simulink model "EHB_speedgoat_R2020a_V1"  (R2020a)
settings: Solver=FixedStepDiscrete  StartTime=0.0  StopTime=inf  FixedStep=0.001  RelTol=1e-3  EnableMultiTasking=on
model workspace (MAT data in the model file):
  A : Simulink.Signal (value not decoded)
  B : Simulink.Signal (value not decoded)
  C : Simulink.Signal (value not decoded)
  D : Simulink.Signal (value not decoded)
  E : Simulink.Signal (value not decoded)
  calin = [-9.96 -7.98 -5.98 -3.99 -1.994 0 1.995 3.992 5.99 7.98 9.97]
  calout = [-10 -8 -6 -4 -2 0 2 4 6 8 10]
symbols that are objects in the model workspace (value not decoded): C, D
undefined symbols (not defined in the file): Com1, none, ts_IO612
libraries: simulink x1436, xpcethercatlib x1223, yisutbxlib_utilities x256, xpcutilitieslib x156, hdlsllib x145, canmsglib x46, speedgoatlib_IO602_4 x11, speedgoatlib_IO611 x7, slrttcplib x4, CanManageLib x3, slrtlib x3, xpcseriallib x2
(part 23 of 30)

== system EHB_speedgoat_R2020a_V1/保留/TIF_06/YS4020_M_1/YS4020_M/FIU_CH1 ==
  FIU_SetCH1 : Inport
  "Bit Unpacking " : xpcutilitieslib/Bit Unpacking   SignExtend=on  MaskBitPatterns={[0],[1],[2],[3]}  MaskPackDataType=uint8  MaskPackDataSize=[1]  MaskUnpackDataTypes={'boolean','boolean','boolean','boolean'}  MaskUnpackDataSizes={[1],[1],[1],[1]}
      settings: SourceProductBaseCode=XP
  Bus Creator : BusCreator  Inputs=4
  Protect : Subsystem
  CH1_Out : Outport
  wires:
  FIU_SetCH1/1 -> "Bit Unpacking "/1
  Protect/3(COM_Out) -> Bus Creator/3  "COM_Out"
  Protect/2(KL31_Out) -> Bus Creator/2  "KL31_Out"
  Protect/1(KL30_Out) -> Bus Creator/1  "KL30_Out"
  Protect/4(Open_Out) -> Bus Creator/4  "Open_Out"
  "Bit Unpacking "/1 -> Protect/1(KL30_In)
  "Bit Unpacking "/2 -> Protect/2(KL31_In)
  "Bit Unpacking "/3 -> Protect/3(COM_In)
  "Bit Unpacking "/4 -> Protect/4(Open_In)
  Bus Creator/1 -> CH1_Out/1

== system EHB_speedgoat_R2020a_V1/保留/TIF_06/YS4020_M_1/YS4020_M/FIU_CH10 ==
  FIU_SetCH10 : Inport
  "Bit Unpacking " : xpcutilitieslib/Bit Unpacking   SignExtend=on  MaskBitPatterns={[0],[1],[2],[3]}  MaskPackDataType=uint8  MaskPackDataSize=[1]  MaskUnpackDataTypes={'boolean','boolean','boolean','boolean'}  MaskUnpackDataSizes={[1],[1],[1],[1]}
      settings: SourceProductBaseCode=XP
  Bus Creator : BusCreator  Inputs=4
  Protect : Subsystem
  CH10_Out : Outport
  wires:
  Bus Creator/1 -> CH10_Out/1
  "Bit Unpacking "/4 -> Protect/4(Open_In)
  "Bit Unpacking "/3 -> Protect/3(COM_In)
  "Bit Unpacking "/2 -> Protect/2(KL31_In)
  "Bit Unpacking "/1 -> Protect/1(KL30_In)
  Protect/4(Open_Out) -> Bus Creator/4  "Open_Out"
  Protect/1(KL30_Out) -> Bus Creator/1  "KL30_Out"
  Protect/2(KL31_Out) -> Bus Creator/2  "KL31_Out"
  Protect/3(COM_Out) -> Bus Creator/3  "COM_Out"
  FIU_SetCH10/1 -> "Bit Unpacking "/1

== system EHB_speedgoat_R2020a_V1/保留/TIF_06/YS4020_M_1/YS4020_M/FIU_CH11 ==
  FIU_SetCH1 : Inport
  "Bit Unpacking " : xpcutilitieslib/Bit Unpacking   SignExtend=on  MaskBitPatterns={[0],[1],[2],[3]}  MaskPackDataType=uint8  MaskPackDataSize=[1]  MaskUnpackDataTypes={'boolean','boolean','boolean','boolean'}  MaskUnpackDataSizes={[1],[1],[1],[1]}
      settings: SourceProductBaseCode=XP
  Bus Creator : BusCreator  Inputs=4
  Protect : Subsystem
  CH1_Out : Outport
  wires:
  Bus Creator/1 -> CH1_Out/1
  "Bit Unpacking "/4 -> Protect/4(Open_In)
  "Bit Unpacking "/3 -> Protect/3(COM_In)
  "Bit Unpacking "/2 -> Protect/2(KL31_In)
  "Bit Unpacking "/1 -> Protect/1(KL30_In)
  Protect/4(Open_Out) -> Bus Creator/4  "Open_Out"
  Protect/1(KL30_Out) -> Bus Creator/1  "KL30_Out"
  Protect/2(KL31_Out) -> Bus Creator/2  "KL31_Out"
  Protect/3(COM_Out) -> Bus Creator/3  "COM_Out"
  FIU_SetCH1/1 -> "Bit Unpacking "/1

== system EHB_speedgoat_R2020a_V1/保留/TIF_06/YS4020_M_1/YS4020_M/FIU_CH12 ==
  FIU_SetCH10 : Inport
  "Bit Unpacking " : xpcutilitieslib/Bit Unpacking   SignExtend=on  MaskBitPatterns={[0],[1],[2],[3]}  MaskPackDataType=uint8  MaskPackDataSize=[1]  MaskUnpackDataTypes={'boolean','boolean','boolean','boolean'}  MaskUnpackDataSizes={[1],[1],[1],[1]}
      settings: SourceProductBaseCode=XP
  Bus Creator : BusCreator  Inputs=4
  Protect : Subsystem
  CH10_Out : Outport
  wires:
  FIU_SetCH10/1 -> "Bit Unpacking "/1
  Protect/3(COM_Out) -> Bus Creator/3  "COM_Out"
  Protect/2(KL31_Out) -> Bus Creator/2  "KL31_Out"
  Protect/1(KL30_Out) -> Bus Creator/1  "KL30_Out"
  Protect/4(Open_Out) -> Bus Creator/4  "Open_Out"
  "Bit Unpacking "/1 -> Protect/1(KL30_In)
  "Bit Unpacking "/2 -> Protect/2(KL31_In)
  "Bit Unpacking "/3 -> Protect/3(COM_In)
  "Bit Unpacking "/4 -> Protect/4(Open_In)
  Bus Creator/1 -> CH10_Out/1

== system EHB_speedgoat_R2020a_V1/保留/TIF_06/YS4020_M_1/YS4020_M/FIU_CH13 ==
  FIU_SetCH2 : Inport
  "Bit Unpacking " : xpcutilitieslib/Bit Unpacking   SignExtend=on  MaskBitPatterns={[0],[1],[2],[3]}  MaskPackDataType=uint8  MaskPackDataSize=[1]  MaskUnpackDataTypes={'boolean','boolean','boolean','boolean'}  MaskUnpackDataSizes={[1],[1],[1],[1]}
      settings: SourceProductBaseCode=XP
  Bus Creator : BusCreator  Inputs=4
  Protect : Subsystem
  CH2_Out : Outport
  wires:
  FIU_SetCH2/1 -> "Bit Unpacking "/1
  Protect/3(COM_Out) -> Bus Creator/3  "COM_Out"
  Protect/2(KL31_Out) -> Bus Creator/2  "KL31_Out"
  Protect/1(KL30_Out) -> Bus Creator/1  "KL30_Out"
  Protect/4(Open_Out) -> Bus Creator/4  "Open_Out"
  "Bit Unpacking "/1 -> Protect/1(KL30_In)
  "Bit Unpacking "/2 -> Protect/2(KL31_In)
  "Bit Unpacking "/3 -> Protect/3(COM_In)
  "Bit Unpacking "/4 -> Protect/4(Open_In)
  Bus Creator/1 -> CH2_Out/1

== system EHB_speedgoat_R2020a_V1/保留/TIF_06/YS4020_M_1/YS4020_M/FIU_CH14 ==
  FIU_SetCH3 : Inport
  "Bit Unpacking " : xpcutilitieslib/Bit Unpacking   SignExtend=on  MaskBitPatterns={[0],[1],[2],[3]}  MaskPackDataType=uint8  MaskPackDataSize=[1]  MaskUnpackDataTypes={'boolean','boolean','boolean','boolean'}  MaskUnpackDataSizes={[1],[1],[1],[1]}
      settings: SourceProductBaseCode=XP
  Bus Creator : BusCreator  Inputs=4
  Protect : Subsystem
  CH3_Out : Outport
  wires:
  Bus Creator/1 -> CH3_Out/1
  "Bit Unpacking "/4 -> Protect/4(Open_In)
  "Bit Unpacking "/3 -> Protect/3(COM_In)
  "Bit Unpacking "/2 -> Protect/2(KL31_In)
  "Bit Unpacking "/1 -> Protect/1(KL30_In)
  Protect/4(Open_Out) -> Bus Creator/4  "Open_Out"
  Protect/1(KL30_Out) -> Bus Creator/1  "KL30_Out"
  Protect/2(KL31_Out) -> Bus Creator/2  "KL31_Out"
  Protect/3(COM_Out) -> Bus Creator/3  "COM_Out"
  FIU_SetCH3/1 -> "Bit Unpacking "/1

== system EHB_speedgoat_R2020a_V1/保留/TIF_06/YS4020_M_1/YS4020_M/FIU_CH15 ==
  FIU_SetCH4 : Inport
  "Bit Unpacking " : xpcutilitieslib/Bit Unpacking   SignExtend=on  MaskBitPatterns={[0],[1],[2],[3]}  MaskPackDataType=uint8  MaskPackDataSize=[1]  MaskUnpackDataTypes={'boolean','boolean','boolean','boolean'}  MaskUnpackDataSizes={[1],[1],[1],[1]}
      settings: SourceProductBaseCode=XP
  Bus Creator : BusCreator  Inputs=4
  Protect : Subsystem
  CH4_Out : Outport
  wires:
  FIU_SetCH4/1 -> "Bit Unpacking "/1
  Protect/3(COM_Out) -> Bus Creator/3  "COM_Out"
  Protect/2(KL31_Out) -> Bus Creator/2  "KL31_Out"
  Protect/1(KL30_Out) -> Bus Creator/1  "KL30_Out"
  Protect/4(Open_Out) -> Bus Creator/4  "Open_Out"
  "Bit Unpacking "/1 -> Protect/1(KL30_In)
  "Bit Unpacking "/2 -> Protect/2(KL31_In)
  "Bit Unpacking "/3 -> Protect/3(COM_In)
  "Bit Unpacking "/4 -> Protect/4(Open_In)
  Bus Creator/1 -> CH4_Out/1

== system EHB_speedgoat_R2020a_V1/保留/TIF_06/YS4020_M_1/YS4020_M/FIU_CH16 ==
  FIU_SetCH5 : Inport
  "Bit Unpacking " : xpcutilitieslib/Bit Unpacking   SignExtend=on  MaskBitPatterns={[0],[1],[2],[3]}  MaskPackDataType=uint8  MaskPackDataSize=[1]  MaskUnpackDataTypes={'boolean','boolean','boolean','boolean'}  MaskUnpackDataSizes={[1],[1],[1],[1]}
      settings: SourceProductBaseCode=XP
  Bus Creator : BusCreator  Inputs=4
  Protect : Subsystem
  CH5_Out : Outport
  wires:
  Bus Creator/1 -> CH5_Out/1
  "Bit Unpacking "/4 -> Protect/4(Open_In)
  "Bit Unpacking "/3 -> Protect/3(COM_In)
  "Bit Unpacking "/2 -> Protect/2(KL31_In)
  "Bit Unpacking "/1 -> Protect/1(KL30_In)
  Protect/4(Open_Out) -> Bus Creator/4  "Open_Out"
  Protect/1(KL30_Out) -> Bus Creator/1  "KL30_Out"
  Protect/2(KL31_Out) -> Bus Creator/2  "KL31_Out"
  Protect/3(COM_Out) -> Bus Creator/3  "COM_Out"
  FIU_SetCH5/1 -> "Bit Unpacking "/1

== system EHB_speedgoat_R2020a_V1/保留/TIF_06/YS4020_M_1/YS4020_M/FIU_CH17 ==
  FIU_SetCH6 : Inport
  "Bit Unpacking " : xpcutilitieslib/Bit Unpacking   SignExtend=on  MaskBitPatterns={[0],[1],[2],[3]}  MaskPackDataType=uint8  MaskPackDataSize=[1]  MaskUnpackDataTypes={'boolean','boolean','boolean','boolean'}  MaskUnpackDataSizes={[1],[1],[1],[1]}
      settings: SourceProductBaseCode=XP
  Bus Creator : BusCreator  Inputs=4
  Protect : Subsystem
  CH6_Out : Outport
  wires:
  FIU_SetCH6/1 -> "Bit Unpacking "/1
  Protect/3(COM_Out) -> Bus Creator/3  "COM_Out"
  Protect/2(KL31_Out) -> Bus Creator/2  "KL31_Out"
  Protect/1(KL30_Out) -> Bus Creator/1  "KL30_Out"
  Protect/4(Open_Out) -> Bus Creator/4  "Open_Out"
  "Bit Unpacking "/1 -> Protect/1(KL30_In)
  "Bit Unpacking "/2 -> Protect/2(KL31_In)
  "Bit Unpacking "/3 -> Protect/3(COM_In)
  "Bit Unpacking "/4 -> Protect/4(Open_In)
  Bus Creator/1 -> CH6_Out/1

== system EHB_speedgoat_R2020a_V1/保留/TIF_06/YS4020_M_1/YS4020_M/FIU_CH18 ==
  FIU_SetCH7 : Inport
  "Bit Unpacking " : xpcutilitieslib/Bit Unpacking   SignExtend=on  MaskBitPatterns={[0],[1],[2],[3]}  MaskPackDataType=uint8  MaskPackDataSize=[1]  MaskUnpackDataTypes={'boolean','boolean','boolean','boolean'}  MaskUnpackDataSizes={[1],[1],[1],[1]}
      settings: SourceProductBaseCode=XP
  Bus Creator : BusCreator  Inputs=4
  Protect : Subsystem
  CH7_Out : Outport
  wires:
  Bus Creator/1 -> CH7_Out/1
  "Bit Unpacking "/4 -> Protect/4(Open_In)
  "Bit Unpacking "/3 -> Protect/3(COM_In)
  "Bit Unpacking "/2 -> Protect/2(KL31_In)
  "Bit Unpacking "/1 -> Protect/1(KL30_In)
  Protect/4(Open_Out) -> Bus Creator/4  "Open_Out"
  Protect/1(KL30_Out) -> Bus Creator/1  "KL30_Out"
  Protect/2(KL31_Out) -> Bus Creator/2  "KL31_Out"
  Protect/3(COM_Out) -> Bus Creator/3  "COM_Out"
  FIU_SetCH7/1 -> "Bit Unpacking "/1

== system EHB_speedgoat_R2020a_V1/保留/TIF_06/YS4020_M_1/YS4020_M/FIU_CH19 ==
  FIU_SetCH8 : Inport
  "Bit Unpacking " : xpcutilitieslib/Bit Unpacking   SignExtend=on  MaskBitPatterns={[0],[1],[2],[3]}  MaskPackDataType=uint8  MaskPackDataSize=[1]  MaskUnpackDataTypes={'boolean','boolean','boolean','boolean'}  MaskUnpackDataSizes={[1],[1],[1],[1]}
      settings: SourceProductBaseCode=XP
  Bus Creator : BusCreator  Inputs=4
  Protect : Subsystem
  CH8_Out : Outport
  wires:
  FIU_SetCH8/1 -> "Bit Unpacking "/1
  Protect/3(COM_Out) -> Bus Creator/3  "COM_Out"
  Protect/2(KL31_Out) -> Bus Creator/2  "KL31_Out"
  Protect/1(KL30_Out) -> Bus Creator/1  "KL30_Out"
  Protect/4(Open_Out) -> Bus Creator/4  "Open_Out"
  "Bit Unpacking "/1 -> Protect/1(KL30_In)
  "Bit Unpacking "/2 -> Protect/2(KL31_In)
  "Bit Unpacking "/3 -> Protect/3(COM_In)
  "Bit Unpacking "/4 -> Protect/4(Open_In)
  Bus Creator/1 -> CH8_Out/1

== system EHB_speedgoat_R2020a_V1/保留/TIF_06/YS4020_M_1/YS4020_M/FIU_CH2 ==
  FIU_SetCH2 : Inport
  "Bit Unpacking " : xpcutilitieslib/Bit Unpacking   SignExtend=on  MaskBitPatterns={[0],[1],[2],[3]}  MaskPackDataType=uint8  MaskPackDataSize=[1]  MaskUnpackDataTypes={'boolean','boolean','boolean','boolean'}  MaskUnpackDataSizes={[1],[1],[1],[1]}
      settings: SourceProductBaseCode=XP
  Bus Creator : BusCreator  Inputs=4
  Protect : Subsystem
  CH2_Out : Outport
  wires:
  Bus Creator/1 -> CH2_Out/1
  "Bit Unpacking "/4 -> Protect/4(Open_In)
  "Bit Unpacking "/3 -> Protect/3(COM_In)
  "Bit Unpacking "/2 -> Protect/2(KL31_In)
  "Bit Unpacking "/1 -> Protect/1(KL30_In)
  Protect/4(Open_Out) -> Bus Creator/4  "Open_Out"
  Protect/1(KL30_Out) -> Bus Creator/1  "KL30_Out"
  Protect/2(KL31_Out) -> Bus Creator/2  "KL31_Out"
  Protect/3(COM_Out) -> Bus Creator/3  "COM_Out"
  FIU_SetCH2/1 -> "Bit Unpacking "/1

== system EHB_speedgoat_R2020a_V1/保留/TIF_06/YS4020_M_1/YS4020_M/FIU_CH20 ==
  FIU_SetCH9 : Inport
  "Bit Unpacking " : xpcutilitieslib/Bit Unpacking   SignExtend=on  MaskBitPatterns={[0],[1],[2],[3]}  MaskPackDataType=uint8  MaskPackDataSize=[1]  MaskUnpackDataTypes={'boolean','boolean','boolean','boolean'}  MaskUnpackDataSizes={[1],[1],[1],[1]}
      settings: SourceProductBaseCode=XP
  Bus Creator : BusCreator  Inputs=4
  Protect : Subsystem
  CH9_Out : Outport
  wires:
  Bus Creator/1 -> CH9_Out/1
  "Bit Unpacking "/4 -> Protect/4(Open_In)
  "Bit Unpacking "/3 -> Protect/3(COM_In)
  "Bit Unpacking "/2 -> Protect/2(KL31_In)
  "Bit Unpacking "/1 -> Protect/1(KL30_In)
  Protect/4(Open_Out) -> Bus Creator/4  "Open_Out"
  Protect/1(KL30_Out) -> Bus Creator/1  "KL30_Out"
  Protect/2(KL31_Out) -> Bus Creator/2  "KL31_Out"
  Protect/3(COM_Out) -> Bus Creator/3  "COM_Out"
  FIU_SetCH9/1 -> "Bit Unpacking "/1

== system EHB_speedgoat_R2020a_V1/保留/TIF_06/YS4020_M_1/YS4020_M/FIU_CH3 ==
  FIU_SetCH3 : Inport
  "Bit Unpacking " : xpcutilitieslib/Bit Unpacking   SignExtend=on  MaskBitPatterns={[0],[1],[2],[3]}  MaskPackDataType=uint8  MaskPackDataSize=[1]  MaskUnpackDataTypes={'boolean','boolean','boolean','boolean'}  MaskUnpackDataSizes={[1],[1],[1],[1]}
      settings: SourceProductBaseCode=XP
  Bus Creator : BusCreator  Inputs=4
  Protect : Subsystem
  CH3_Out : Outport
  wires:
  FIU_SetCH3/1 -> "Bit Unpacking "/1
  Protect/3(COM_Out) -> Bus Creator/3  "COM_Out"
  Protect/2(KL31_Out) -> Bus Creator/2  "KL31_Out"
  Protect/1(KL30_Out) -> Bus Creator/1  "KL30_Out"
  Protect/4(Open_Out) -> Bus Creator/4  "Open_Out"
  "Bit Unpacking "/1 -> Protect/1(KL30_In)
  "Bit Unpacking "/2 -> Protect/2(KL31_In)
  "Bit Unpacking "/3 -> Protect/3(COM_In)
  "Bit Unpacking "/4 -> Protect/4(Open_In)
  Bus Creator/1 -> CH3_Out/1

== system EHB_speedgoat_R2020a_V1/保留/TIF_06/YS4020_M_1/YS4020_M/FIU_CH4 ==
  FIU_SetCH4 : Inport
  "Bit Unpacking " : xpcutilitieslib/Bit Unpacking   SignExtend=on  MaskBitPatterns={[0],[1],[2],[3]}  MaskPackDataType=uint8  MaskPackDataSize=[1]  MaskUnpackDataTypes={'boolean','boolean','boolean','boolean'}  MaskUnpackDataSizes={[1],[1],[1],[1]}
      settings: SourceProductBaseCode=XP
  Bus Creator : BusCreator  Inputs=4
  Protect : Subsystem
  CH4_Out : Outport
  wires:
  Bus Creator/1 -> CH4_Out/1
  "Bit Unpacking "/4 -> Protect/4(Open_In)
  "Bit Unpacking "/3 -> Protect/3(COM_In)
  "Bit Unpacking "/2 -> Protect/2(KL31_In)
  "Bit Unpacking "/1 -> Protect/1(KL30_In)
  Protect/4(Open_Out) -> Bus Creator/4  "Open_Out"
  Protect/1(KL30_Out) -> Bus Creator/1  "KL30_Out"
  Protect/2(KL31_Out) -> Bus Creator/2  "KL31_Out"
  Protect/3(COM_Out) -> Bus Creator/3  "COM_Out"
  FIU_SetCH4/1 -> "Bit Unpacking "/1

== system EHB_speedgoat_R2020a_V1/保留/TIF_06/YS4020_M_1/YS4020_M/FIU_CH5 ==
  FIU_SetCH5 : Inport
  "Bit Unpacking " : xpcutilitieslib/Bit Unpacking   SignExtend=on  MaskBitPatterns={[0],[1],[2],[3]}  MaskPackDataType=uint8  MaskPackDataSize=[1]  MaskUnpackDataTypes={'boolean','boolean','boolean','boolean'}  MaskUnpackDataSizes={[1],[1],[1],[1]}
      settings: SourceProductBaseCode=XP
  Bus Creator : BusCreator  Inputs=4
  Protect : Subsystem
  CH5_Out : Outport
  wires:
  FIU_SetCH5/1 -> "Bit Unpacking "/1
  Protect/3(COM_Out) -> Bus Creator/3  "COM_Out"
  Protect/2(KL31_Out) -> Bus Creator/2  "KL31_Out"
  Protect/1(KL30_Out) -> Bus Creator/1  "KL30_Out"
  Protect/4(Open_Out) -> Bus Creator/4  "Open_Out"
  "Bit Unpacking "/1 -> Protect/1(KL30_In)
  "Bit Unpacking "/2 -> Protect/2(KL31_In)
  "Bit Unpacking "/3 -> Protect/3(COM_In)
  "Bit Unpacking "/4 -> Protect/4(Open_In)
  Bus Creator/1 -> CH5_Out/1

== system EHB_speedgoat_R2020a_V1/保留/TIF_06/YS4020_M_1/YS4020_M/FIU_CH6 ==
  FIU_SetCH6 : Inport
  "Bit Unpacking " : xpcutilitieslib/Bit Unpacking   SignExtend=on  MaskBitPatterns={[0],[1],[2],[3]}  MaskPackDataType=uint8  MaskPackDataSize=[1]  MaskUnpackDataTypes={'boolean','boolean','boolean','boolean'}  MaskUnpackDataSizes={[1],[1],[1],[1]}
      settings: SourceProductBaseCode=XP
  Bus Creator : BusCreator  Inputs=4
  Protect : Subsystem
  CH6_Out : Outport
  wires:
  Bus Creator/1 -> CH6_Out/1
  "Bit Unpacking "/4 -> Protect/4(Open_In)
  "Bit Unpacking "/3 -> Protect/3(COM_In)
  "Bit Unpacking "/2 -> Protect/2(KL31_In)
  "Bit Unpacking "/1 -> Protect/1(KL30_In)
  Protect/4(Open_Out) -> Bus Creator/4  "Open_Out"
  Protect/1(KL30_Out) -> Bus Creator/1  "KL30_Out"
  Protect/2(KL31_Out) -> Bus Creator/2  "KL31_Out"
  Protect/3(COM_Out) -> Bus Creator/3  "COM_Out"
  FIU_SetCH6/1 -> "Bit Unpacking "/1

== system EHB_speedgoat_R2020a_V1/保留/TIF_06/YS4020_M_1/YS4020_M/FIU_CH7 ==
  FIU_SetCH7 : Inport
  "Bit Unpacking " : xpcutilitieslib/Bit Unpacking   SignExtend=on  MaskBitPatterns={[0],[1],[2],[3]}  MaskPackDataType=uint8  MaskPackDataSize=[1]  MaskUnpackDataTypes={'boolean','boolean','boolean','boolean'}  MaskUnpackDataSizes={[1],[1],[1],[1]}
      settings: SourceProductBaseCode=XP
  Bus Creator : BusCreator  Inputs=4
  Protect : Subsystem
  CH7_Out : Outport
  wires:
  FIU_SetCH7/1 -> "Bit Unpacking "/1
  Protect/3(COM_Out) -> Bus Creator/3  "COM_Out"
  Protect/2(KL31_Out) -> Bus Creator/2  "KL31_Out"
  Protect/1(KL30_Out) -> Bus Creator/1  "KL30_Out"
  Protect/4(Open_Out) -> Bus Creator/4  "Open_Out"
  "Bit Unpacking "/1 -> Protect/1(KL30_In)
  "Bit Unpacking "/2 -> Protect/2(KL31_In)
  "Bit Unpacking "/3 -> Protect/3(COM_In)
  "Bit Unpacking "/4 -> Protect/4(Open_In)
  Bus Creator/1 -> CH7_Out/1

== system EHB_speedgoat_R2020a_V1/保留/TIF_06/YS4020_M_1/YS4020_M/FIU_CH8 ==
  FIU_SetCH8 : Inport
  "Bit Unpacking " : xpcutilitieslib/Bit Unpacking   SignExtend=on  MaskBitPatterns={[0],[1],[2],[3]}  MaskPackDataType=uint8  MaskPackDataSize=[1]  MaskUnpackDataTypes={'boolean','boolean','boolean','boolean'}  MaskUnpackDataSizes={[1],[1],[1],[1]}
      settings: SourceProductBaseCode=XP
  Bus Creator : BusCreator  Inputs=4
  Protect : Subsystem
  CH8_Out : Outport
  wires:
  Bus Creator/1 -> CH8_Out/1
  "Bit Unpacking "/4 -> Protect/4(Open_In)
  "Bit Unpacking "/3 -> Protect/3(COM_In)
  "Bit Unpacking "/2 -> Protect/2(KL31_In)
  "Bit Unpacking "/1 -> Protect/1(KL30_In)
  Protect/4(Open_Out) -> Bus Creator/4  "Open_Out"
  Protect/1(KL30_Out) -> Bus Creator/1  "KL30_Out"
  Protect/2(KL31_Out) -> Bus Creator/2  "KL31_Out"
  Protect/3(COM_Out) -> Bus Creator/3  "COM_Out"
  FIU_SetCH8/1 -> "Bit Unpacking "/1

== system EHB_speedgoat_R2020a_V1/保留/TIF_06/YS4020_M_1/YS4020_M/FIU_CH9 ==
  FIU_SetCH9 : Inport
  "Bit Unpacking " : xpcutilitieslib/Bit Unpacking   SignExtend=on  MaskBitPatterns={[0],[1],[2],[3]}  MaskPackDataType=uint8  MaskPackDataSize=[1]  MaskUnpackDataTypes={'boolean','boolean','boolean','boolean'}  MaskUnpackDataSizes={[1],[1],[1],[1]}
      settings: SourceProductBaseCode=XP
  Bus Creator : BusCreator  Inputs=4
  Protect : Subsystem
  CH9_Out : Outport
  wires:
  FIU_SetCH9/1 -> "Bit Unpacking "/1
  Protect/3(COM_Out) -> Bus Creator/3  "COM_Out"
  Protect/2(KL31_Out) -> Bus Creator/2  "KL31_Out"
  Protect/1(KL30_Out) -> Bus Creator/1  "KL30_Out"
  Protect/4(Open_Out) -> Bus Creator/4  "Open_Out"
  "Bit Unpacking "/1 -> Protect/1(KL30_In)
  "Bit Unpacking "/2 -> Protect/2(KL31_In)
  "Bit Unpacking "/3 -> Protect/3(COM_In)
  "Bit Unpacking "/4 -> Protect/4(Open_In)
  Bus Creator/1 -> CH9_Out/1

== system EHB_speedgoat_R2020a_V1/保留/TIF_06/YS4020_M_1/YS4020_M/FIU_MsgSend ==
  YS4020_M : Inport
  Enable : EnablePort
  Bus Selector : BusSelector  OutputSignals=CH1_Out.KL30_Out,CH1_Out.KL31_Out,CH1_Out.COM_Out,CH1_Out.Open_Out,CH2_Out.KL30_Out,CH2_Out.KL31_Out,CH2_Out.COM_Out,CH2_Out.Open_Out,CH3_Out.KL30_Out,CH3_Out.KL31_Out,CH3_Out.COM_Out,CH3_Out.Open_Out,CH4_Out.KL30_Out,CH4_Out.KL31_Out,CH4_Out.COM_Out,CH4_Out.Open_Out,CH5_Out.KL30_Out,CH5_Out.KL31_Out,CH5_Out.COM_Out,CH5_Out.Open_Out,CH6_Out.KL30_Out,CH6_Out.KL31_Out,CH6_Out.COM_Out,CH6_Out.Open_Out,CH7_Out.KL30_Out,CH7_Out.KL31_Out,CH7_Out.COM_Out,CH7_Out.Open_Out,CH8_Out.KL30_Out,CH8_Out.KL31_Out,CH8_Out.COM_Out,CH8_Out.Open_Out,CH9_Out.KL30_Out,CH9_Out.KL31_Out,CH9_Out.COM_Out,CH9_Out.Open_Out,CH10_Out.KL30_Out,CH10_Out.KL31_Out,CH10_Out.COM_Out,CH10_Out.Open_Out,PassWord,YS4020_M_Slot
  CAN Pack8 : canmsglib/CAN Pack  MsgList=(none)  MsgName=FIUStsSet  MsgIDType=Standard (11-bit identifier)  MsgIdentifier=1553  MsgLength=8  Remote=off  ApplyMinMax=off  BusOutput=on  SignalInfo={ 'CH10_COM', '62', '1', 'BE', 'unsigned', 'Standard', '0', '1', '0', '0', '1'; 'CH10_KL30', '60', '1', 'BE', 'unsigned', 'Standard', '0', '1', '0', '0', '1'; 'CH10_KL31', '61', '1', 'BE', 'unsigned', 'Standard', '0', '1', '0', '0', '1'; 'CH10_Open', '63', '1', 'BE', 'unsigned', 'Standard', '0', '1', '0', '0', '1'; 'CH1_COM', '26', '1', 'BE', 'unsigned', 'Standard', '0', '1', '0', '0', '1'; 'CH1_KL30', '24', '1', 'BE', 'unsigned', 'Standard', '0', '1', '0', '0', '1'; 'CH1_KL31', '25', '1', 'BE', 'unsigned', 'Standard', '0', '1', '0', '0', '1'; 'CH1_Open', '27', '1', 'BE', 'unsigned', 'Standard', '0', '1', '0', '0', '1'; 'CH2_COM', '30', '1', 'BE', 'unsigned', 'Standard', '0', '1', '0', '0', '1'; 'CH2_KL30', '28', '1', 'BE', 'unsigned', 'Standard', '0', '1', '0', '0', '1'; 'CH2_KL31', '29', '1', 'BE', 'unsigned', 'Standard', '0', '1', '0', '0', '1'; 'CH2_Open', '31', '1', 'BE', 'unsigned', 'Standard', '0', '1', '0', '0', '1'; 'CH3_COM', '34', '1', 'BE', 'unsigned', 'Standard', '0', '1', '0', '0', '1'; 'CH3_KL30', '32', '1', 'BE', 'unsigned', 'Standard', '0', '1', '0', '0', '1'; 'CH3_KL31', '33', '1', 'BE', 'unsigned', 'Standard', '0', '1', '0', '0', '1'; 'CH3_Open', '35', '1', 'BE', 'unsigned', 'Standard', '0', '1', '0', '0', '1'; 'CH4_COM', '38', '1', 'BE', 'unsigned', 'Standard', '0', '1', '0', '0', '1'; 'CH4_KL30', '36', '1', 'BE', 'unsigned', 'Standard', '0', '1', '0', '0', '1'; 'CH4_KL31', '37', '1', 'BE', 'unsigned', 'Standard', '0', '1', '0', '0', '1'; 'CH4_Open', '39', '1', 'BE', 'unsigned', 'Standard', '0', '1', '0', '0', '1'; 'CH5_COM', '42', '1', 'BE', 'unsigned', 'Standard', '0', '1', '0', '0', '1'; 'CH5_KL30', '40', '1', 'BE', 'unsigned', 'Standard', '0', '1', '0', '0', '1'; 'CH5_KL31', '41', '1', 'BE', 'unsigned', 'Standard', '0', '1', '0', '0', '1'; 'CH5_Open', '43', '1', 'BE', 'unsigned', 'Standard', '0', '1', '0', '0', '1'; 'CH6_COM', '46', '1', 'BE', 'unsigned', 'Standard', '0', '1', '0', '0', '1'; 'CH6_KL30', '44', '1', 'BE', 'unsigned', 'Standard', '0', '1', '0', '0', '1'; 'CH6_KL31', '45', '1', 'BE', 'unsigned', 'Standard', '0', '1', '0', '0', '1'; 'CH6_Open', '47', '1', 'BE', 'unsigned', 'Standard', '0', '1', '0', '0', '1'; 'CH7_COM', '50', '1', 'BE', 'unsigned', 'Standard', '0', '1', '0', '0', '1'; 'CH7_KL30', '48', '1', 'BE', 'unsigned', 'Standard', '0', '1', '0', '0', '1'; 'CH7_KL31', '49', '1', 'BE', 'unsigned', 'Standard', '0', '1', '0', '0', '1'; 'CH7_Open', '51', '1', 'BE', 'unsigned', 'Standard', '0', '1', '0', '0', '1'; 'CH8_COM', '54', '1', 'BE', 'unsigned', 'Standard', '0', '1', '0', '0', '1'; 'CH8_KL30', '52', '1', 'BE', 'unsigned', 'Standard', '0', '1', '0', '0', '1'; 'CH8_KL31', '53', '1', 'BE', 'unsigned', 'Standard', '0', '1', '0', '0', '1'; 'CH8_Open', '55', '1', 'BE', 'unsigned', 'Standard', '0', '1', '0', '0', '1'; 'CH9_COM', '58', '1', 'BE', 'unsigned', 'Standard', '0', '1', '0', '0', '1'; 'CH9_KL30', '56', '1', 'BE', 'unsigned', 'Standard', '0', '1', '0', '0', '1'; 'CH9_KL31', '57', '1', 'BE', 'unsigned', 'Standard', '0', '1', '0', '0', '1'; 'CH9_Open', '59', '1', 'BE', 'unsigned', 'Standard', '0', '1', '0', '0', '1'; 'PassWord', '16', '8', 'BE', 'unsigned', 'Standard', '0', '1', '0', '0', '15'; 'Slot', '0', '4', 'BE', 'unsigned', 'Standard', '0', '1', '0', '0', '15' }
      settings: SourceProductBaseCode=ME,VN  DataFormat=manually specified signals
  CANDataPack_ToUDP : Subsystem
  Output : Outport
  wires:
  [YS4020_M_Slot] -> CAN Pack8/42  "YS4020_M_Slot"
  [CH10_COM] -> CAN Pack8/1  "CH10_COM"
  [CH10_KL30] -> CAN Pack8/2  "CH10_KL30"
  [CH10_KL31] -> CAN Pack8/3  "CH10_KL31"
  [CH10_Open] -> CAN Pack8/4  "CH10_Open"
  [CH1_COM] -> CAN Pack8/5  "CH1_COM"
  [CH1_KL30] -> CAN Pack8/6  "CH1_KL30"
  [CH1_KL31] -> CAN Pack8/7  "CH1_KL31"
  [CH1_Open] -> CAN Pack8/8  "CH1_Open"
  [CH2_COM] -> CAN Pack8/9  "CH2_COM"
  [CH2_KL30] -> CAN Pack8/10  "CH2_KL30"
  [CH2_KL31] -> CAN Pack8/11  "CH2_KL31"
  [CH2_Open] -> CAN Pack8/12  "CH2_Open"
  [CH3_COM] -> CAN Pack8/13  "CH3_COM"
  [CH3_KL30] -> CAN Pack8/14  "CH3_KL30"
  [CH3_KL31] -> CAN Pack8/15  "CH3_KL31"
  [CH3_Open] -> CAN Pack8/16  "CH3_Open"
  [CH4_COM] -> CAN Pack8/17  "CH4_COM"
  [CH4_KL30] -> CAN Pack8/18  "CH4_KL30"
  [CH4_KL31] -> CAN Pack8/19  "CH4_KL31"
  [CH4_Open] -> CAN Pack8/20  "CH4_Open"
  [CH5_COM] -> CAN Pack8/21  "CH5_COM"
  [CH5_KL30] -> CAN Pack8/22  "CH5_KL30"
  [CH5_KL31] -> CAN Pack8/23  "CH5_KL31"
  [CH5_Open] -> CAN Pack8/24  "CH5_Open"
  [CH6_COM] -> CAN Pack8/25  "CH6_COM"
  [CH6_KL30] -> CAN Pack8/26  "CH6_KL30"
  [CH6_KL31] -> CAN Pack8/27  "CH6_KL31"
  [CH6_Open] -> CAN Pack8/28  "CH6_Open"
  [CH7_COM] -> CAN Pack8/29  "CH7_COM"
  [CH7_KL30] -> CAN Pack8/30  "CH7_KL30"
  [CH7_KL31] -> CAN Pack8/31  "CH7_KL31"
  [CH7_Open] -> CAN Pack8/32  "CH7_Open"
  [CH8_COM] -> CAN Pack8/33  "CH8_COM"
  [CH8_KL30] -> CAN Pack8/34  "CH8_KL30"
  [CH8_KL31] -> CAN Pack8/35  "CH8_KL31"
  [CH8_Open] -> CAN Pack8/36  "CH8_Open"
  [CH9_COM] -> CAN Pack8/37  "CH9_COM"
  [CH9_KL30] -> CAN Pack8/38  "CH9_KL30"
  [CH9_KL31] -> CAN Pack8/39  "CH9_KL31"
  [CH9_Open] -> CAN Pack8/40  "CH9_Open"
  [PassWord] -> CAN Pack8/41  "PassWord"
  YS4020_M/1 -> Bus Selector/1
  Bus Selector/1 -> [CH1_KL30]  "<KL30_Out>"
  Bus Selector/2 -> [CH1_KL31]  "<KL31_Out>"
  Bus Selector/3 -> [CH1_COM]  "<COM_Out>"
  Bus Selector/4 -> [CH1_Open]  "<Open_Out>"
  Bus Selector/5 -> [CH2_KL30]  "<KL30_Out>"
  Bus Selector/6 -> [CH2_KL31]  "<KL31_Out>"
  Bus Selector/7 -> [CH2_COM]  "<COM_Out>"
  Bus Selector/8 -> [CH2_Open]  "<Open_Out>"
  Bus Selector/9 -> [CH3_KL30]  "<KL30_Out>"
  Bus Selector/10 -> [CH3_KL31]  "<KL31_Out>"
  Bus Selector/11 -> [CH3_COM]  "<COM_Out>"
  Bus Selector/12 -> [CH3_Open]  "<Open_Out>"
  Bus Selector/13 -> [CH4_KL30]  "<KL30_Out>"
  Bus Selector/14 -> [CH4_KL31]  "<KL31_Out>"
  Bus Selector/15 -> [CH4_COM]  "<COM_Out>"
  Bus Selector/16 -> [CH4_Open]  "<Open_Out>"
  Bus Selector/17 -> [CH5_KL30]  "<KL30_Out>"
  Bus Selector/18 -> [CH5_KL31]  "<KL31_Out>"
  Bus Selector/19 -> [CH5_COM]  "<COM_Out>"
  Bus Selector/20 -> [CH5_Open]  "<Open_Out>"
  Bus Selector/21 -> [CH6_KL30]  "<KL30_Out>"
  Bus Selector/22 -> [CH6_KL31]  "<KL31_Out>"
  Bus Selector/23 -> [CH6_COM]  "<COM_Out>"
  Bus Selector/24 -> [CH6_Open]  "<Open_Out>"
  Bus Selector/25 -> [CH7_KL30]  "<KL30_Out>"
  Bus Selector/26 -> [CH7_KL31]  "<KL31_Out>"
  Bus Selector/27 -> [CH7_COM]  "<COM_Out>"
  Bus Selector/28 -> [CH7_Open]  "<Open_Out>"
  Bus Selector/29 -> [CH8_KL30]  "<KL30_Out>"
  Bus Selector/30 -> [CH8_KL31]  "<KL31_Out>"
  Bus Selector/31 -> [CH8_COM]  "<COM_Out>"
  Bus Selector/32 -> [CH8_Open]  "<Open_Out>"
  Bus Selector/33 -> [CH9_KL30]  "<KL30_Out>"
  Bus Selector/34 -> [CH9_KL31]  "<KL31_Out>"
  Bus Selector/35 -> [CH9_COM]  "<COM_Out>"
  Bus Selector/36 -> [CH9_Open]  "<Open_Out>"
  Bus Selector/37 -> [CH10_KL30]  "<KL30_Out>"
  Bus Selector/38 -> [CH10_KL31]  "<KL31_Out>"
  Bus Selector/39 -> [CH10_COM]  "<COM_Out>"
  Bus Selector/40 -> [CH10_Open]  "<Open_Out>"
  Bus Selector/41 -> [PassWord]  "<PassWord>"
  Bus Selector/42 -> [YS4020_M_Slot]  "<YS4020_M_Slot>"
  CANDataPack_ToUDP/1(Output) -> Output/1
  CAN Pack8/1 -> CANDataPack_ToUDP/1(In1)

== system EHB_speedgoat_R2020a_V1/保留/TIF_06/YS4020_M_1/YS4020_M/FIU_MsgSend1 ==
  YS4020_M : Inport
  Enable : EnablePort
  Bus Selector : BusSelector  OutputSignals=CH1_Out.KL30_Out,CH1_Out.KL31_Out,CH1_Out.COM_Out,CH1_Out.Open_Out,CH2_Out.KL30_Out,CH2_Out.KL31_Out,CH2_Out.COM_Out,CH2_Out.Open_Out,CH3_Out.KL30_Out,CH3_Out.KL31_Out,CH3_Out.COM_Out,CH3_Out.Open_Out,CH4_Out.KL30_Out,CH4_Out.KL31_Out,CH4_Out.COM_Out,CH4_Out.Open_Out,CH5_Out.KL30_Out,CH5_Out.KL31_Out,CH5_Out.COM_Out,CH5_Out.Open_Out,CH6_Out.KL30_Out,CH6_Out.KL31_Out,CH6_Out.COM_Out,CH6_Out.Open_Out,CH7_Out.KL30_Out,CH7_Out.KL31_Out,CH7_Out.COM_Out,CH7_Out.Open_Out,CH8_Out.KL30_Out,CH8_Out.KL31_Out,CH8_Out.COM_Out,CH8_Out.Open_Out,CH9_Out.KL30_Out,CH9_Out.KL31_Out,CH9_Out.COM_Out,CH9_Out.Open_Out,CH10_Out.KL30_Out,CH10_Out.KL31_Out,CH10_Out.COM_Out,CH10_Out.Open_Out,PassWord,YS4020_M_Slot
  CAN Pack8 : canmsglib/CAN Pack  MsgList=(none)  MsgName=FIUStsSet  MsgIDType=Standard (11-bit identifier)  MsgIdentifier=1569  MsgLength=8  Remote=off  ApplyMinMax=off  BusOutput=on  SignalInfo={ 'CH10_COM', '62', '1', 'BE', 'unsigned', 'Standard', '0', '1', '0', '0', '1'; 'CH10_KL30', '60', '1', 'BE', 'unsigned', 'Standard', '0', '1', '0', '0', '1'; 'CH10_KL31', '61', '1', 'BE', 'unsigned', 'Standard', '0', '1', '0', '0', '1'; 'CH10_Open', '63', '1', 'BE', 'unsigned', 'Standard', '0', '1', '0', '0', '1'; 'CH1_COM', '26', '1', 'BE', 'unsigned', 'Standard', '0', '1', '0', '0', '1'; 'CH1_KL30', '24', '1', 'BE', 'unsigned', 'Standard', '0', '1', '0', '0', '1'; 'CH1_KL31', '25', '1', 'BE', 'unsigned', 'Standard', '0', '1', '0', '0', '1'; 'CH1_Open', '27', '1', 'BE', 'unsigned', 'Standard', '0', '1', '0', '0', '1'; 'CH2_COM', '30', '1', 'BE', 'unsigned', 'Standard', '0', '1', '0', '0', '1'; 'CH2_KL30', '28', '1', 'BE', 'unsigned', 'Standard', '0', '1', '0', '0', '1'; 'CH2_KL31', '29', '1', 'BE', 'unsigned', 'Standard', '0', '1', '0', '0', '1'; 'CH2_Open', '31', '1', 'BE', 'unsigned', 'Standard', '0', '1', '0', '0', '1'; 'CH3_COM', '34', '1', 'BE', 'unsigned', 'Standard', '0', '1', '0', '0', '1'; 'CH3_KL30', '32', '1', 'BE', 'unsigned', 'Standard', '0', '1', '0', '0', '1'; 'CH3_KL31', '33', '1', 'BE', 'unsigned', 'Standard', '0', '1', '0', '0', '1'; 'CH3_Open', '35', '1', 'BE', 'unsigned', 'Standard', '0', '1', '0', '0', '1'; 'CH4_COM', '38', '1', 'BE', 'unsigned', 'Standard', '0', '1', '0', '0', '1'; 'CH4_KL30', '36', '1', 'BE', 'unsigned', 'Standard', '0', '1', '0', '0', '1'; 'CH4_KL31', '37', '1', 'BE', 'unsigned', 'Standard', '0', '1', '0', '0', '1'; 'CH4_Open', '39', '1', 'BE', 'unsigned', 'Standard', '0', '1', '0', '0', '1'; 'CH5_COM', '42', '1', 'BE', 'unsigned', 'Standard', '0', '1', '0', '0', '1'; 'CH5_KL30', '40', '1', 'BE', 'unsigned', 'Standard', '0', '1', '0', '0', '1'; 'CH5_KL31', '41', '1', 'BE', 'unsigned', 'Standard', '0', '1', '0', '0', '1'; 'CH5_Open', '43', '1', 'BE', 'unsigned', 'Standard', '0', '1', '0', '0', '1'; 'CH6_COM', '46', '1', 'BE', 'unsigned', 'Standard', '0', '1', '0', '0', '1'; 'CH6_KL30', '44', '1', 'BE', 'unsigned', 'Standard', '0', '1', '0', '0', '1'; 'CH6_KL31', '45', '1', 'BE', 'unsigned', 'Standard', '0', '1', '0', '0', '1'; 'CH6_Open', '47', '1', 'BE', 'unsigned', 'Standard', '0', '1', '0', '0', '1'; 'CH7_COM', '50', '1', 'BE', 'unsigned', 'Standard', '0', '1', '0', '0', '1'; 'CH7_KL30', '48', '1', 'BE', 'unsigned', 'Standard', '0', '1', '0', '0', '1'; 'CH7_KL31', '49', '1', 'BE', 'unsigned', 'Standard', '0', '1', '0', '0', '1'; 'CH7_Open', '51', '1', 'BE', 'unsigned', 'Standard', '0', '1', '0', '0', '1'; 'CH8_COM', '54', '1', 'BE', 'unsigned', 'Standard', '0', '1', '0', '0', '1'; 'CH8_KL30', '52', '1', 'BE', 'unsigned', 'Standard', '0', '1', '0', '0', '1'; 'CH8_KL31', '53', '1', 'BE', 'unsigned', 'Standard', '0', '1', '0', '0', '1'; 'CH8_Open', '55', '1', 'BE', 'unsigned', 'Standard', '0', '1', '0', '0', '1'; 'CH9_COM', '58', '1', 'BE', 'unsigned', 'Standard', '0', '1', '0', '0', '1'; 'CH9_KL30', '56', '1', 'BE', 'unsigned', 'Standard', '0', '1', '0', '0', '1'; 'CH9_KL31', '57', '1', 'BE', 'unsigned', 'Standard', '0', '1', '0', '0', '1'; 'CH9_Open', '59', '1', 'BE', 'unsigned', 'Standard', '0', '1', '0', '0', '1'; 'PassWord', '16', '8', 'BE', 'unsigned', 'Standard', '0', '1', '0', '0', '15'; 'Slot', '0', '4', 'BE', 'unsigned', 'Standard', '0', '1', '0', '0', '15' }
      settings: SourceProductBaseCode=ME,VN  DataFormat=manually specified signals
  CANDataPack_ToUDP : Subsystem
  Output : Outport
  wires:
  YS4020_M/1 -> Bus Selector/1
  [PassWord] -> CAN Pack8/41  "PassWord"
  [CH9_Open] -> CAN Pack8/40  "CH9_Open"
  [CH9_KL31] -> CAN Pack8/39  "CH9_KL31"
  [CH9_KL30] -> CAN Pack8/38  "CH9_KL30"
  [CH9_COM] -> CAN Pack8/37  "CH9_COM"
  [CH8_Open] -> CAN Pack8/36  "CH8_Open"
  [CH8_KL31] -> CAN Pack8/35  "CH8_KL31"
  [CH8_KL30] -> CAN Pack8/34  "CH8_KL30"
  [CH8_COM] -> CAN Pack8/33  "CH8_COM"
  [CH7_Open] -> CAN Pack8/32  "CH7_Open"
  [CH7_KL31] -> CAN Pack8/31  "CH7_KL31"
  [CH7_KL30] -> CAN Pack8/30  "CH7_KL30"
  [CH7_COM] -> CAN Pack8/29  "CH7_COM"
  [CH6_Open] -> CAN Pack8/28  "CH6_Open"
  [CH6_KL31] -> CAN Pack8/27  "CH6_KL31"
  [CH6_KL30] -> CAN Pack8/26  "CH6_KL30"
  [CH6_COM] -> CAN Pack8/25  "CH6_COM"
  [CH5_Open] -> CAN Pack8/24  "CH5_Open"
  [CH5_KL31] -> CAN Pack8/23  "CH5_KL31"
  [CH5_KL30] -> CAN Pack8/22  "CH5_KL30"
  [CH5_COM] -> CAN Pack8/21  "CH5_COM"
  [CH4_Open] -> CAN Pack8/20  "CH4_Open"
  [CH4_KL31] -> CAN Pack8/19  "CH4_KL31"
  [CH4_KL30] -> CAN Pack8/18  "CH4_KL30"
  [CH4_COM] -> CAN Pack8/17  "CH4_COM"
  [CH3_Open] -> CAN Pack8/16  "CH3_Open"
  [CH3_KL31] -> CAN Pack8/15  "CH3_KL31"
  [CH3_KL30] -> CAN Pack8/14  "CH3_KL30"
  [CH3_COM] -> CAN Pack8/13  "CH3_COM"
  [CH2_Open] -> CAN Pack8/12  "CH2_Open"
  [CH2_KL31] -> CAN Pack8/11  "CH2_KL31"
  [CH2_KL30] -> CAN Pack8/10  "CH2_KL30"
  [CH2_COM] -> CAN Pack8/9  "CH2_COM"
  [CH1_Open] -> CAN Pack8/8  "CH1_Open"
  [CH1_KL31] -> CAN Pack8/7  "CH1_KL31"
  [CH1_KL30] -> CAN Pack8/6  "CH1_KL30"
  [CH1_COM] -> CAN Pack8/5  "CH1_COM"
  [CH10_Open] -> CAN Pack8/4  "CH10_Open"
  [CH10_KL31] -> CAN Pack8/3  "CH10_KL31"
  [CH10_KL30] -> CAN Pack8/2  "CH10_KL30"
  [CH10_COM] -> CAN Pack8/1  "CH10_COM"
  [YS4020_M_Slot] -> CAN Pack8/42  "YS4020_M_Slot"
  Bus Selector/1 -> [CH1_KL30]  "<KL30_Out>"
  Bus Selector/2 -> [CH1_KL31]  "<KL31_Out>"
  Bus Selector/3 -> [CH1_COM]  "<COM_Out>"
  Bus Selector/4 -> [CH1_Open]  "<Open_Out>"
  Bus Selector/5 -> [CH2_KL30]  "<KL30_Out>"
  Bus Selector/6 -> [CH2_KL31]  "<KL31_Out>"
  Bus Selector/7 -> [CH2_COM]  "<COM_Out>"
  Bus Selector/8 -> [CH2_Open]  "<Open_Out>"
  Bus Selector/9 -> [CH3_KL30]  "<KL30_Out>"
  Bus Selector/10 -> [CH3_KL31]  "<KL31_Out>"
  Bus Selector/11 -> [CH3_COM]  "<COM_Out>"
  Bus Selector/12 -> [CH3_Open]  "<Open_Out>"
  Bus Selector/13 -> [CH4_KL30]  "<KL30_Out>"
  Bus Selector/14 -> [CH4_KL31]  "<KL31_Out>"
  Bus Selector/15 -> [CH4_COM]  "<COM_Out>"
  Bus Selector/16 -> [CH4_Open]  "<Open_Out>"
  Bus Selector/17 -> [CH5_KL30]  "<KL30_Out>"
  Bus Selector/18 -> [CH5_KL31]  "<KL31_Out>"
  Bus Selector/19 -> [CH5_COM]  "<COM_Out>"
  Bus Selector/20 -> [CH5_Open]  "<Open_Out>"
  Bus Selector/21 -> [CH6_KL30]  "<KL30_Out>"
  Bus Selector/22 -> [CH6_KL31]  "<KL31_Out>"
  Bus Selector/23 -> [CH6_COM]  "<COM_Out>"
  Bus Selector/24 -> [CH6_Open]  "<Open_Out>"
  Bus Selector/25 -> [CH7_KL30]  "<KL30_Out>"
  Bus Selector/26 -> [CH7_KL31]  "<KL31_Out>"
  Bus Selector/27 -> [CH7_COM]  "<COM_Out>"
  Bus Selector/28 -> [CH7_Open]  "<Open_Out>"
  Bus Selector/29 -> [CH8_KL30]  "<KL30_Out>"
  Bus Selector/30 -> [CH8_KL31]  "<KL31_Out>"
  Bus Selector/31 -> [CH8_COM]  "<COM_Out>"
  Bus Selector/32 -> [CH8_Open]  "<Open_Out>"
  Bus Selector/33 -> [CH9_KL30]  "<KL30_Out>"
  Bus Selector/34 -> [CH9_KL31]  "<KL31_Out>"
  Bus Selector/35 -> [CH9_COM]  "<COM_Out>"
  Bus Selector/36 -> [CH9_Open]  "<Open_Out>"
  Bus Selector/37 -> [CH10_KL30]  "<KL30_Out>"
  Bus Selector/38 -> [CH10_KL31]  "<KL31_Out>"
  Bus Selector/39 -> [CH10_COM]  "<COM_Out>"
  Bus Selector/40 -> [CH10_Open]  "<Open_Out>"
  Bus Selector/41 -> [PassWord]  "<PassWord>"
  Bus Selector/42 -> [YS4020_M_Slot]  "<YS4020_M_Slot>"
  CAN Pack8/1 -> CANDataPack_ToUDP/1(In1)
  CANDataPack_ToUDP/1(Output) -> Output/1

== system EHB_speedgoat_R2020a_V1/保留/TIF_06/YS4020_M_1/YS4020_M/YS4020_M_Ctrl_Trigger ==
  CH1_10 : Inport
  Bitwise Operator : simulink/Logic and Bit Operations/Bitwise Operator  logicop=OR  UseBitMask=off  BitMask=bin2dec('11011001')  BitMaskRealWorld=Stored Integer
  Demux : Demux  Outputs=10
  Detect Change : simulink/Logic and Bit Operations/Detect Change  vinit=0  OutDataTypeStr=boolean
  Mux : Mux  Inputs=10
  YS4020_M_CtrlTrigger : Outport
  wires:
  Detect Change/1 -> Bitwise Operator/1
  Mux/1 -> Detect Change/1
  Bitwise Operator/1 -> YS4020_M_CtrlTrigger/1
  CH1_10/1 -> Demux/1
  Demux/1 -> Mux/1
  Demux/2 -> Mux/2
  Demux/3 -> Mux/3
  Demux/4 -> Mux/4
  Demux/5 -> Mux/5
  Demux/6 -> Mux/6
  Demux/7 -> Mux/7
  Demux/8 -> Mux/8
  Demux/9 -> Mux/9
  Demux/10 -> Mux/10

== system EHB_speedgoat_R2020a_V1/保留/TIF_06/YS4020_M_1/YS4020_M/YS4020_M_Ctrl_Trigger1 ==
  CH11_20 : Inport
  Bitwise Operator : simulink/Logic and Bit Operations/Bitwise Operator  logicop=OR  UseBitMask=off  BitMask=bin2dec('11011001')  BitMaskRealWorld=Stored Integer
  Demux1 : Demux  Outputs=10
  Detect Change : simulink/Logic and Bit Operations/Detect Change  vinit=0  OutDataTypeStr=boolean
  Mux : Mux  Inputs=10
  YS4020_M_CtrlTrigger : Outport
  wires:
  CH11_20/1 -> Demux1/1
  Demux1/10 -> Mux/10
  Demux1/9 -> Mux/9
  Demux1/8 -> Mux/8
  Demux1/7 -> Mux/7
  Demux1/6 -> Mux/6
  Demux1/5 -> Mux/5
  Demux1/4 -> Mux/4
  Demux1/3 -> Mux/3
  Demux1/2 -> Mux/2
  Demux1/1 -> Mux/1
  Bitwise Operator/1 -> YS4020_M_CtrlTrigger/1
  Mux/1 -> Detect Change/1
  Detect Change/1 -> Bitwise Operator/1

== system EHB_speedgoat_R2020a_V1/保留/YS4008/YS4008_M_1/YS4008_M/FIU_CH1 ==
  FIU_SetCH1 : Inport
  Bit Unpacking 1 : xpcutilitieslib/Bit Unpacking   SignExtend=on  MaskBitPatterns={[0],[1],[2],[3]}  MaskPackDataType=uint8  MaskPackDataSize=[1]  MaskUnpackDataTypes={'boolean','boolean','boolean','boolean'}  MaskUnpackDataSizes={[1],[1],[1],[1]}
      settings: SourceProductBaseCode=XP
  Bus Creator : BusCreator  Inputs=4
  Protect : Subsystem
  CH1_Out : Outport
  wires:
  FIU_SetCH1/1 -> Bit Unpacking 1/1
  Protect/3(COM_Out) -> Bus Creator/3  "COM_Out"
  Protect/2(KL31_Out) -> Bus Creator/2  "KL31_Out"
  Protect/1(KL30_Out) -> Bus Creator/1  "KL30_Out"
  Protect/4(Open_Out) -> Bus Creator/4  "Open_Out"
  Bit Unpacking 1/1 -> Protect/1(KL30_In)
  Bit Unpacking 1/2 -> Protect/2(KL31_In)
  Bit Unpacking 1/3 -> Protect/3(COM_In)
  Bit Unpacking 1/4 -> Protect/4(Open_In)
  Bus Creator/1 -> CH1_Out/1

== system EHB_speedgoat_R2020a_V1/保留/YS4008/YS4008_M_1/YS4008_M/FIU_CH2 ==
  FIU_SetCH2 : Inport
  Bit Unpacking 1 : xpcutilitieslib/Bit Unpacking   SignExtend=on  MaskBitPatterns={[0],[1],[2],[3]}  MaskPackDataType=uint8  MaskPackDataSize=[1]  MaskUnpackDataTypes={'boolean','boolean','boolean','boolean'}  MaskUnpackDataSizes={[1],[1],[1],[1]}
      settings: SourceProductBaseCode=XP
  Bus Creator : BusCreator  Inputs=4
  Protect : Subsystem
  CH2_Out : Outport
  wires:
  Bus Creator/1 -> CH2_Out/1
  Bit Unpacking 1/4 -> Protect/4(Open_In)
  Bit Unpacking 1/3 -> Protect/3(COM_In)
  Bit Unpacking 1/2 -> Protect/2(KL31_In)
  Bit Unpacking 1/1 -> Protect/1(KL30_In)
  Protect/4(Open_Out) -> Bus Creator/4  "Open_Out"
  Protect/1(KL30_Out) -> Bus Creator/1  "KL30_Out"
  Protect/2(KL31_Out) -> Bus Creator/2  "KL31_Out"
  Protect/3(COM_Out) -> Bus Creator/3  "COM_Out"
  FIU_SetCH2/1 -> Bit Unpacking 1/1

== system EHB_speedgoat_R2020a_V1/保留/YS4008/YS4008_M_1/YS4008_M/FIU_CH3 ==
  FIU_SetCH3 : Inport
  Bit Unpacking 1 : xpcutilitieslib/Bit Unpacking   SignExtend=on  MaskBitPatterns={[0],[1],[2],[3]}  MaskPackDataType=uint8  MaskPackDataSize=[1]  MaskUnpackDataTypes={'boolean','boolean','boolean','boolean'}  MaskUnpackDataSizes={[1],[1],[1],[1]}
      settings: SourceProductBaseCode=XP
  Bus Creator : BusCreator  Inputs=4
  Protect : Subsystem
  CH3_Out : Outport
  wires:
  FIU_SetCH3/1 -> Bit Unpacking 1/1
  Protect/3(COM_Out) -> Bus Creator/3  "COM_Out"
  Protect/2(KL31_Out) -> Bus Creator/2  "KL31_Out"
  Protect/1(KL30_Out) -> Bus Creator/1  "KL30_Out"
  Protect/4(Open_Out) -> Bus Creator/4  "Open_Out"
  Bit Unpacking 1/1 -> Protect/1(KL30_In)
  Bit Unpacking 1/2 -> Protect/2(KL31_In)
  Bit Unpacking 1/3 -> Protect/3(COM_In)
  Bit Unpacking 1/4 -> Protect/4(Open_In)
  Bus Creator/1 -> CH3_Out/1

== system EHB_speedgoat_R2020a_V1/保留/YS4008/YS4008_M_1/YS4008_M/FIU_CH4 ==
  FIU_SetCH4 : Inport
  Bit Unpacking 1 : xpcutilitieslib/Bit Unpacking   SignExtend=on  MaskBitPatterns={[0],[1],[2],[3]}  MaskPackDataType=uint8  MaskPackDataSize=[1]  MaskUnpackDataTypes={'boolean','boolean','boolean','boolean'}  MaskUnpackDataSizes={[1],[1],[1],[1]}
      settings: SourceProductBaseCode=XP
  Bus Creator : BusCreator  Inputs=4
  Protect : Subsystem
  CH4_Out : Outport
  wires:
  Bus Creator/1 -> CH4_Out/1
  Bit Unpacking 1/4 -> Protect/4(Open_In)
  Bit Unpacking 1/3 -> Protect/3(COM_In)
  Bit Unpacking 1/2 -> Protect/2(KL31_In)
  Bit Unpacking 1/1 -> Protect/1(KL30_In)
  Protect/4(Open_Out) -> Bus Creator/4  "Open_Out"
  Protect/1(KL30_Out) -> Bus Creator/1  "KL30_Out"
  Protect/2(KL31_Out) -> Bus Creator/2  "KL31_Out"
  Protect/3(COM_Out) -> Bus Creator/3  "COM_Out"
  FIU_SetCH4/1 -> Bit Unpacking 1/1

== system EHB_speedgoat_R2020a_V1/保留/YS4008/YS4008_M_1/YS4008_M/FIU_CH5 ==
  FIU_SetCH5 : Inport
  Bit Unpacking 1 : xpcutilitieslib/Bit Unpacking   SignExtend=on  MaskBitPatterns={[0],[1],[2],[3]}  MaskPackDataType=uint8  MaskPackDataSize=[1]  MaskUnpackDataTypes={'boolean','boolean','boolean','boolean'}  MaskUnpackDataSizes={[1],[1],[1],[1]}
      settings: SourceProductBaseCode=XP
  Bus Creator : BusCreator  Inputs=4
  Protect : Subsystem
  CH5_Out : Outport
  wires:
  FIU_SetCH5/1 -> Bit Unpacking 1/1
  Protect/3(COM_Out) -> Bus Creator/3  "COM_Out"
  Protect/2(KL31_Out) -> Bus Creator/2  "KL31_Out"
  Protect/1(KL30_Out) -> Bus Creator/1  "KL30_Out"
  Protect/4(Open_Out) -> Bus Creator/4  "Open_Out"
  Bit Unpacking 1/1 -> Protect/1(KL30_In)
  Bit Unpacking 1/2 -> Protect/2(KL31_In)
  Bit Unpacking 1/3 -> Protect/3(COM_In)
  Bit Unpacking 1/4 -> Protect/4(Open_In)
  Bus Creator/1 -> CH5_Out/1

== system EHB_speedgoat_R2020a_V1/保留/YS4008/YS4008_M_1/YS4008_M/FIU_CH6 ==
  FIU_SetCH6 : Inport
  Bit Unpacking 1 : xpcutilitieslib/Bit Unpacking   SignExtend=on  MaskBitPatterns={[0],[1],[2],[3]}  MaskPackDataType=uint8  MaskPackDataSize=[1]  MaskUnpackDataTypes={'boolean','boolean','boolean','boolean'}  MaskUnpackDataSizes={[1],[1],[1],[1]}
      settings: SourceProductBaseCode=XP
  Bus Creator : BusCreator  Inputs=4
  Protect : Subsystem
  CH6_Out : Outport
  wires:
  Bus Creator/1 -> CH6_Out/1
  Bit Unpacking 1/4 -> Protect/4(Open_In)
  Bit Unpacking 1/3 -> Protect/3(COM_In)
  Bit Unpacking 1/2 -> Protect/2(KL31_In)
  Bit Unpacking 1/1 -> Protect/1(KL30_In)
  Protect/4(Open_Out) -> Bus Creator/4  "Open_Out"
  Protect/1(KL30_Out) -> Bus Creator/1  "KL30_Out"
  Protect/2(KL31_Out) -> Bus Creator/2  "KL31_Out"
  Protect/3(COM_Out) -> Bus Creator/3  "COM_Out"
  FIU_SetCH6/1 -> Bit Unpacking 1/1

== system EHB_speedgoat_R2020a_V1/保留/YS4008/YS4008_M_1/YS4008_M/FIU_CH7 ==
  FIU_SetCH7 : Inport
  Bit Unpacking 1 : xpcutilitieslib/Bit Unpacking   SignExtend=on  MaskBitPatterns={[0],[1],[2],[3]}  MaskPackDataType=uint8  MaskPackDataSize=[1]  MaskUnpackDataTypes={'boolean','boolean','boolean','boolean'}  MaskUnpackDataSizes={[1],[1],[1],[1]}
      settings: SourceProductBaseCode=XP
  Bus Creator : BusCreator  Inputs=4
  Protect : Subsystem
  CH7_Out : Outport
  wires:
  FIU_SetCH7/1 -> Bit Unpacking 1/1
  Protect/3(COM_Out) -> Bus Creator/3  "COM_Out"
  Protect/2(KL31_Out) -> Bus Creator/2  "KL31_Out"
  Protect/1(KL30_Out) -> Bus Creator/1  "KL30_Out"
  Protect/4(Open_Out) -> Bus Creator/4  "Open_Out"
  Bit Unpacking 1/1 -> Protect/1(KL30_In)
  Bit Unpacking 1/2 -> Protect/2(KL31_In)
  Bit Unpacking 1/3 -> Protect/3(COM_In)
  Bit Unpacking 1/4 -> Protect/4(Open_In)
  Bus Creator/1 -> CH7_Out/1

== system EHB_speedgoat_R2020a_V1/保留/YS4008/YS4008_M_1/YS4008_M/FIU_CH8 ==
  FIU_SetCH8 : Inport
  Bit Unpacking 1 : xpcutilitieslib/Bit Unpacking   SignExtend=on  MaskBitPatterns={[0],[1],[2],[3]}  MaskPackDataType=uint8  MaskPackDataSize=[1]  MaskUnpackDataTypes={'boolean','boolean','boolean','boolean'}  MaskUnpackDataSizes={[1],[1],[1],[1]}
      settings: SourceProductBaseCode=XP
  Bus Creator : BusCreator  Inputs=4
  Protect : Subsystem
  CH8_Out : Outport
  wires:
  Bus Creator/1 -> CH8_Out/1
  Bit Unpacking 1/4 -> Protect/4(Open_In)
  Bit Unpacking 1/3 -> Protect/3(COM_In)
  Bit Unpacking 1/2 -> Protect/2(KL31_In)
  Bit Unpacking 1/1 -> Protect/1(KL30_In)
  Protect/4(Open_Out) -> Bus Creator/4  "Open_Out"
  Protect/1(KL30_Out) -> Bus Creator/1  "KL30_Out"
  Protect/2(KL31_Out) -> Bus Creator/2  "KL31_Out"
  Protect/3(COM_Out) -> Bus Creator/3  "COM_Out"
  FIU_SetCH8/1 -> Bit Unpacking 1/1

== system EHB_speedgoat_R2020a_V1/保留/YS4008/YS4008_M_1/YS4008_M/FIU_MsgSend ==
  YS4008_M : Inport
  Enable : EnablePort
  Bus Selector : BusSelector  OutputSignals=CH1_Out.KL30_Out,CH1_Out.KL31_Out,CH1_Out.COM_Out,CH1_Out.Open_Out,CH2_Out.KL30_Out,CH2_Out.KL31_Out,CH2_Out.COM_Out,CH2_Out.Open_Out,CH3_Out.KL30_Out,CH3_Out.KL31_Out,CH3_Out.COM_Out,CH3_Out.Open_Out,CH4_Out.KL30_Out,CH4_Out.KL31_Out,CH4_Out.COM_Out,CH4_Out.Open_Out,CH5_Out.KL30_Out,CH5_Out.KL31_Out,CH5_Out.COM_Out,CH5_Out.Open_Out,CH6_Out.KL30_Out,CH6_Out.KL31_Out,CH6_Out.COM_Out,CH6_Out.Open_Out,CH7_Out.KL30_Out,CH7_Out.KL31_Out,CH7_Out.COM_Out,CH7_Out.Open_Out,CH8_Out.KL30_Out,CH8_Out.KL31_Out,CH8_Out.COM_Out,CH8_Out.Open_Out,PassWord,Rack,Slot
  CAN Pack8 : canmsglib/CAN Pack  MsgList=(none)  MsgName=FIUStsSet  MsgIDType=Standard (11-bit identifier)  MsgIdentifier=1665  MsgLength=8  Remote=off  ApplyMinMax=off  BusOutput=on  SignalInfo={ 'CH1_COM', '26', '1', 'BE', 'unsigned', 'Standard', '0', '1', '0', '0', '1'; 'CH1_KL30', '24', '1', 'BE', 'unsigned', 'Standard', '0', '1', '0', '0', '1'; 'CH1_KL31', '25', '1', 'BE', 'unsigned', 'Standard', '0', '1', '0', '0', '1'; 'CH1_Open', '27', '1', 'BE', 'unsigned', 'Standard', '0', '1', '0', '0', '1'; 'CH2_COM', '30', '1', 'BE', 'unsigned', 'Standard', '0', '1', '0', '0', '1'; 'CH2_KL30', '28', '1', 'BE', 'unsigned', 'Standard', '0', '1', '0', '0', '1'; 'CH2_KL31', '29', '1', 'BE', 'unsigned', 'Standard', '0', '1', '0', '0', '1'; 'CH2_Open', '31', '1', 'BE', 'unsigned', 'Standard', '0', '1', '0', '0', '1'; 'CH3_COM', '34', '1', 'BE', 'unsigned', 'Standard', '0', '1', '0', '0', '1'; 'CH3_KL30', '32', '1', 'BE', 'unsigned', 'Standard', '0', '1', '0', '0', '1'; 'CH3_KL31', '33', '1', 'BE', 'unsigned', 'Standard', '0', '1', '0', '0', '1'; 'CH3_Open', '35', '1', 'BE', 'unsigned', 'Standard', '0', '1', '0', '0', '1'; 'CH4_COM', '38', '1', 'BE', 'unsigned', 'Standard', '0', '1', '0', '0', '1'; 'CH4_KL30', '36', '1', 'BE', 'unsigned', 'Standard', '0', '1', '0', '0', '1'; 'CH4_KL31', '37', '1', 'BE', 'unsigned', 'Standard', '0', '1', '0', '0', '1'; 'CH4_Open', '39', '1', 'BE', 'unsigned', 'Standard', '0', '1', '0', '0', '1'; 'CH5_COM', '42', '1', 'BE', 'unsigned', 'Standard', '0', '1', '0', '0', '1'; 'CH5_KL30', '40', '1', 'BE', 'unsigned', 'Standard', '0', '1', '0', '0', '1'; 'CH5_KL31', '41', '1', 'BE', 'unsigned', 'Standard', '0', '1', '0', '0', '1'; 'CH5_Open', '43', '1', 'BE', 'unsigned', 'Standard', '0', '1', '0', '0', '1'; 'CH6_COM', '46', '1', 'BE', 'unsigned', 'Standard', '0', '1', '0', '0', '1'; 'CH6_KL30', '44', '1', 'BE', 'unsigned', 'Standard', '0', '1', '0', '0', '1'; 'CH6_KL31', '45', '1', 'BE', 'unsigned', 'Standard', '0', '1', '0', '0', '1'; 'CH6_Open', '47', '1', 'BE', 'unsigned', 'Standard', '0', '1', '0', '0', '1'; 'CH7_COM', '50', '1', 'BE', 'unsigned', 'Standard', '0', '1', '0', '0', '1'; 'CH7_KL30', '48', '1', 'BE', 'unsigned', 'Standard', '0', '1', '0', '0', '1'; 'CH7_KL31', '49', '1', 'BE', 'unsigned', 'Standard', '0', '1', '0', '0', '1'; 'CH7_Open', '51', '1', 'BE', 'unsigned', 'Standard', '0', '1', '0', '0', '1'; 'CH8_COM', '54', '1', 'BE', 'unsigned', 'Standard', '0', '1', '0', '0', '1'; 'CH8_KL30', '52', '1', 'BE', 'unsigned', 'Standard', '0', '1', '0', '0', '1'; 'CH8_KL31', '53', '1', 'BE', 'unsigned', 'Standard', '0', '1', '0', '0', '1'; 'CH8_Open', '55', '1', 'BE', 'unsigned', 'Standard', '0', '1', '0', '0', '1'; 'Password', '16', '8', 'BE', 'unsigned', 'Standard', '0', '1', '0', '0', '15'; 'Rack', '0', '4', 'BE', 'signed', 'Standard', '0', '1', '0', '-Inf', 'Inf'; 'Slot', '4', '4', 'BE', 'signed', 'Standard', '0', '1', '0', '-Inf', 'Inf' }
      settings: SourceProductBaseCode=XP,ME,VN  DataFormat=manually specified signals
  CANDataPack_ToUDP : Subsystem
  Output : Outport
  wires:
  YS4008_M/1 -> Bus Selector/1
  [CH1_COM] -> CAN Pack8/1  "CH1_COM"
  [CH1_KL30] -> CAN Pack8/2  "CH1_KL30"
  [CH1_KL31] -> CAN Pack8/3  "CH1_KL31"
  [CH1_Open] -> CAN Pack8/4  "CH1_Open"
  [CH2_COM] -> CAN Pack8/5  "CH2_COM"
  [CH2_KL30] -> CAN Pack8/6  "CH2_KL30"
  [CH2_KL31] -> CAN Pack8/7  "CH2_KL31"
  [CH2_Open] -> CAN Pack8/8  "CH2_Open"
  [CH3_COM] -> CAN Pack8/9  "CH3_COM"
  [CH3_KL30] -> CAN Pack8/10  "CH3_KL30"
  [CH3_KL31] -> CAN Pack8/11  "CH3_KL31"
  [CH3_Open] -> CAN Pack8/12  "CH3_Open"
  [CH4_COM] -> CAN Pack8/13  "CH4_COM"
  [CH4_KL30] -> CAN Pack8/14  "CH4_KL30"
  [CH4_KL31] -> CAN Pack8/15  "CH4_KL31"
  [CH4_Open] -> CAN Pack8/16  "CH4_Open"
  [CH5_COM] -> CAN Pack8/17  "CH5_COM"
  [CH5_KL30] -> CAN Pack8/18  "CH5_KL30"
  [CH5_KL31] -> CAN Pack8/19  "CH5_KL31"
  [CH5_Open] -> CAN Pack8/20  "CH5_Open"
  [CH6_COM] -> CAN Pack8/21  "CH6_COM"
  [CH6_KL30] -> CAN Pack8/22  "CH6_KL30"
  [CH6_KL31] -> CAN Pack8/23  "CH6_KL31"
  [CH6_Open] -> CAN Pack8/24  "CH6_Open"
  [CH7_COM] -> CAN Pack8/25  "CH7_COM"
  [CH7_KL30] -> CAN Pack8/26  "CH7_KL30"
  [CH7_KL31] -> CAN Pack8/27  "CH7_KL31"
  [CH7_Open] -> CAN Pack8/28  "CH7_Open"
  [CH8_COM] -> CAN Pack8/29  "CH8_COM"
  [CH8_KL30] -> CAN Pack8/30  "CH8_KL30"
  [CH8_KL31] -> CAN Pack8/31  "CH8_KL31"
  [CH8_Open] -> CAN Pack8/32  "CH8_Open"
  [PassWord] -> CAN Pack8/33  "PassWord"
  Bus Selector/33 -> [PassWord]  "<PassWord>"
  Bus Selector/9 -> [CH3_KL30]  "<KL30_Out>"
  Bus Selector/10 -> [CH3_KL31]  "<KL31_Out>"
  Bus Selector/11 -> [CH3_COM]  "<COM_Out>"
  Bus Selector/12 -> [CH3_Open]  "<Open_Out>"
  Bus Selector/13 -> [CH4_KL30]  "<KL30_Out>"
  Bus Selector/14 -> [CH4_KL31]  "<KL31_Out>"
  Bus Selector/15 -> [CH4_COM]  "<COM_Out>"
  Bus Selector/16 -> [CH4_Open]  "<Open_Out>"
  Bus Selector/17 -> [CH5_KL30]  "<KL30_Out>"
  Bus Selector/18 -> [CH5_KL31]  "<KL31_Out>"
  Bus Selector/19 -> [CH5_COM]  "<COM_Out>"
  Bus Selector/20 -> [CH5_Open]  "<Open_Out>"
  Bus Selector/21 -> [CH6_KL30]  "<KL30_Out>"
  Bus Selector/22 -> [CH6_KL31]  "<KL31_Out>"
  Bus Selector/23 -> [CH6_COM]  "<COM_Out>"
  Bus Selector/24 -> [CH6_Open]  "<Open_Out>"
  Bus Selector/25 -> [CH7_KL30]  "<KL30_Out>"
  Bus Selector/26 -> [CH7_KL31]  "<KL31_Out>"
  Bus Selector/27 -> [CH7_COM]  "<COM_Out>"
  Bus Selector/28 -> [CH7_Open]  "<Open_Out>"
  Bus Selector/29 -> [CH8_KL30]  "<KL30_Out>"
  Bus Selector/30 -> [CH8_KL31]  "<KL31_Out>"
  Bus Selector/31 -> [CH8_COM]  "<COM_Out>"
  Bus Selector/32 -> [CH8_Open]  "<Open_Out>"
  Bus Selector/1 -> [CH1_KL30]  "<KL30_Out>"
  Bus Selector/2 -> [CH1_KL31]  "<KL31_Out>"
  Bus Selector/3 -> [CH1_COM]  "<COM_Out>"
  Bus Selector/4 -> [CH1_Open]  "<Open_Out>"
  Bus Selector/5 -> [CH2_KL30]  "<KL30_Out>"
  Bus Selector/6 -> [CH2_KL31]  "<KL31_Out>"
  Bus Selector/7 -> [CH2_COM]  "<COM_Out>"
  Bus Selector/8 -> [CH2_Open]  "<Open_Out>"
  [Rack] -> CAN Pack8/34  "Rack"
  [Slot] -> CAN Pack8/35  "Slot"
  Bus Selector/34 -> [Rack]  "<Rack>"
  Bus Selector/35 -> [Slot]  "<Slot>"
  CAN Pack8/1 -> CANDataPack_ToUDP/1(In1)
  CANDataPack_ToUDP/1(Output) -> Output/1

== system EHB_speedgoat_R2020a_V1/保留/YS4008/YS4008_M_1/YS4008_M/YS4008_M_Ctrl_Trigger ==
  YS4008_M : Inport
  Bitwise Operator : simulink/Logic and Bit Operations/Bitwise Operator  logicop=OR  UseBitMask=off  BitMask=bin2dec('11011001')  BitMaskRealWorld=Stored Integer
  Bus Selector : BusSelector  OutputSignals=FIU_SetCH1,FIU_SetCH2,FIU_SetCH3,FIU_SetCH4,FIU_SetCH5,FIU_SetCH6,FIU_SetCH7,FIU_SetCH8
  Detect Change : simulink/Logic and Bit Operations/Detect Change  vinit=0  OutDataTypeStr=boolean
  Mux : Mux  Inputs=8
  YS4008_M_CtrlTrigger : Outport
  wires:
  Detect Change/1 -> Bitwise Operator/1
  Mux/1 -> Detect Change/1
  Bitwise Operator/1 -> YS4008_M_CtrlTrigger/1
  YS4008_M/1 -> Bus Selector/1
  Bus Selector/1 -> Mux/1  "<FIU_SetCH1>"
  Bus Selector/2 -> Mux/2  "<FIU_SetCH2>"
  Bus Selector/3 -> Mux/3  "<FIU_SetCH3>"
  Bus Selector/4 -> Mux/4  "<FIU_SetCH4>"
  Bus Selector/5 -> Mux/5  "<FIU_SetCH5>"
  Bus Selector/6 -> Mux/6  "<FIU_SetCH6>"
  Bus Selector/7 -> Mux/7  "<FIU_SetCH7>"
  Bus Selector/8 -> Mux/8  "<FIU_SetCH8>"

== system EHB_speedgoat_R2020a_V1/保留/YS4008/YS4008_M_2/YS4008_M/FIU_CH1 ==
  FIU_SetCH1 : Inport
  Bit Unpacking 1 : xpcutilitieslib/Bit Unpacking   SignExtend=on  MaskBitPatterns={[0],[1],[2],[3]}  MaskPackDataType=uint8  MaskPackDataSize=[1]  MaskUnpackDataTypes={'boolean','boolean','boolean','boolean'}  MaskUnpackDataSizes={[1],[1],[1],[1]}
      settings: SourceProductBaseCode=XP
  Bus Creator : BusCreator  Inputs=4
  Protect : Subsystem
  CH1_Out : Outport
  wires:
  FIU_SetCH1/1 -> Bit Unpacking 1/1
  Protect/3(COM_Out) -> Bus Creator/3  "COM_Out"
  Protect/2(KL31_Out) -> Bus Creator/2  "KL31_Out"
  Protect/1(KL30_Out) -> Bus Creator/1  "KL30_Out"
  Protect/4(Open_Out) -> Bus Creator/4  "Open_Out"
  Bit Unpacking 1/1 -> Protect/1(KL30_In)
  Bit Unpacking 1/2 -> Protect/2(KL31_In)
  Bit Unpacking 1/3 -> Protect/3(COM_In)
  Bit Unpacking 1/4 -> Protect/4(Open_In)
  Bus Creator/1 -> CH1_Out/1

== system EHB_speedgoat_R2020a_V1/保留/YS4008/YS4008_M_2/YS4008_M/FIU_CH2 ==
  FIU_SetCH2 : Inport
  Bit Unpacking 1 : xpcutilitieslib/Bit Unpacking   SignExtend=on  MaskBitPatterns={[0],[1],[2],[3]}  MaskPackDataType=uint8  MaskPackDataSize=[1]  MaskUnpackDataTypes={'boolean','boolean','boolean','boolean'}  MaskUnpackDataSizes={[1],[1],[1],[1]}
      settings: SourceProductBaseCode=XP
  Bus Creator : BusCreator  Inputs=4
  Protect : Subsystem
  CH2_Out : Outport
  wires:
  Bus Creator/1 -> CH2_Out/1
  Bit Unpacking 1/4 -> Protect/4(Open_In)
  Bit Unpacking 1/3 -> Protect/3(COM_In)
  Bit Unpacking 1/2 -> Protect/2(KL31_In)
  Bit Unpacking 1/1 -> Protect/1(KL30_In)
  Protect/4(Open_Out) -> Bus Creator/4  "Open_Out"
  Protect/1(KL30_Out) -> Bus Creator/1  "KL30_Out"
  Protect/2(KL31_Out) -> Bus Creator/2  "KL31_Out"
  Protect/3(COM_Out) -> Bus Creator/3  "COM_Out"
  FIU_SetCH2/1 -> Bit Unpacking 1/1

== system EHB_speedgoat_R2020a_V1/保留/YS4008/YS4008_M_2/YS4008_M/FIU_CH3 ==
  FIU_SetCH3 : Inport
  Bit Unpacking 1 : xpcutilitieslib/Bit Unpacking   SignExtend=on  MaskBitPatterns={[0],[1],[2],[3]}  MaskPackDataType=uint8  MaskPackDataSize=[1]  MaskUnpackDataTypes={'boolean','boolean','boolean','boolean'}  MaskUnpackDataSizes={[1],[1],[1],[1]}
      settings: SourceProductBaseCode=XP
  Bus Creator : BusCreator  Inputs=4
  Protect : Subsystem
  CH3_Out : Outport
  wires:
  FIU_SetCH3/1 -> Bit Unpacking 1/1
  Protect/3(COM_Out) -> Bus Creator/3  "COM_Out"
  Protect/2(KL31_Out) -> Bus Creator/2  "KL31_Out"
  Protect/1(KL30_Out) -> Bus Creator/1  "KL30_Out"
  Protect/4(Open_Out) -> Bus Creator/4  "Open_Out"
  Bit Unpacking 1/1 -> Protect/1(KL30_In)
  Bit Unpacking 1/2 -> Protect/2(KL31_In)
  Bit Unpacking 1/3 -> Protect/3(COM_In)
  Bit Unpacking 1/4 -> Protect/4(Open_In)
  Bus Creator/1 -> CH3_Out/1
